simulink model "sistema_realimentado_PI"  (Simulink 7.7)
settings: Solver=ode3  StartTime=0.0  StopTime=20  FixedStep=0.01  RelTol=1e-3
libraries: simulink x1
settings Model: Creator=juen  LastModifiedBy=juen
settings DataIOCC: LimitDataPoints=off

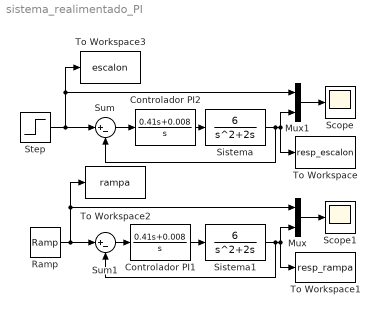
== system sistema_realimentado_PI ==
  Controlador PI1 : TransferFcn  Numerator=[0.41 0.008]  Denominator=[1 0]
  Controlador PI2 : TransferFcn  Numerator=[0.41 0.008]  Denominator=[1 0]
  Mux : Mux  Inputs=2
  Mux1 : Mux  Inputs=2
  Ramp : simulink/Sources/Ramp  SystemSampleTime=-1  slope=1  start=0  X0=0
  Scope : Scope
      settings: TimeRange=50  YMin=1.0003  YMax=1.0009
  Scope1 : Scope
  Sistema : TransferFcn  Numerator=[6]  Denominator=[1 2 0]
  Sistema1 : TransferFcn  Numerator=[6]  Denominator=[1 2 0]
  Step : Step  SampleTime=0
  Sum : Sum  Inputs=|+-
  Sum1 : Sum  Inputs=|+-
  To Workspace : ToWorkspace  VariableName=resp_escalon  SampleTime=-1  SaveFormat=Structure With Time
  To Workspace1 : ToWorkspace  VariableName=resp_rampa  SampleTime=-1  SaveFormat=Structure With Time
  To Workspace2 : ToWorkspace  VariableName=rampa  SampleTime=-1  SaveFormat=Structure With Time
  To Workspace3 : ToWorkspace  VariableName=escalon  SampleTime=-1  SaveFormat=Structure With Time
  wires:
  Sistema/1 -> To Workspace/1, Mux1/2, Sum/2
  Controlador PI2/1 -> Sistema/1
  Step/1 -> Sum/1, To Workspace3/1, Mux1/1
  Sum/1 -> Controlador PI2/1
  Sistema1/1 -> To Workspace1/1, Mux/2, Sum1/2
  Controlador PI1/1 -> Sistema1/1
  Ramp/1 -> Sum1/1, Mux/1, To Workspace2/1
  Sum1/1 -> Controlador PI1/1
  Mux/1 -> Scope1/1
  Mux1/1 -> Scope/1
